simulink model "Project_template"  (R2014b)
settings: Solver=ode23tb  StartTime=0.0  StopTime=600  RelTol=1e-6  AbsTol=1e-6
values from neighbouring files (symbols this model uses):
  k = 1    [testfile.m]
  K_I = 0.03    [engine_sim.m]
  K_p = 0.002    [engine_sim.m]
undefined symbols (not defined in the file or in its folder): a_0, a_1, a_2, AFs, AirStep, alpha_REF_manual, alphaEND, alphaINI, alphaST, Boost_control, C_2, C_d, c_fi, c_fr_0, c_r1, c_r2, dp_thrREF, gamma_air, KiDriver, KpDriver, KpThr, KpWg, n_0, n_1, n_2, n_cyl, N_e_manual, N_e_step, n_ig_ch, n_r, NEND, NeST, Newton, NINI, p_amb, pedEND, pedINI, pedPos_manual, pedST, q_LHV, R_air, r_c, R_exh, Raphson, rho_air, rTurb, t_0, T_0, T_amb, T_hat_bef_thr, T_hat_im, T_ic, T_t, tau_d_bc, tau_th, TiThr, TiWg, V_d, V_D, V_em ... (+10)
libraries: simulink x1
(part 1 of 2)
settings Model: ExtModeTrigMode=oneshot  ExtModeArmWhenConnect=off  ExtModeAutoUpdateStatusClock=off  Creator=peran  LastModifiedBy=nicgr354
settings DataIOCC: LimitDataPoints=off  SignalLoggingSaveFormat=ModelDataLogs  SignalLoggingName=sigsOut
settings OptimizationCC: BlockReduction=off  BooleanDataType=off  UseDivisionForNetSlopeComputation=off  ExpressionDepthLimit=2147483647  InitFltsAndDblsToZero=on  SimCompilerOptimization=off
settings DebuggingCC: SaveWithParameterizedLinksMsg=none  UnderspecifiedInitializationDetection=Classic  MergeDetectMultiDrivingBlocksExec=none  SignalResolutionControl=TryResolveAllWithWarning  SolverPrmCheckMsg=none  MultiTaskDSMMsg=warning  MultiTaskCondExecSysMsg=none  FcnCallInpInsideContextMsg=UseLocalSettings  FrameProcessingCompatibilityMsg=error  AllowSymbolicDim=off  StateNameClashWarn=warning
settings HardwareCC: TargetUnknown=on
settings RTWCC: RTWCompilerOptimization=off
settings GRTTargetCC: TargetFcnLib=ansi_tfl_tmw.mat  ModelReferenceCompliant=off  CombineOutputUpdateFcns=off  MatFileLogging=off  GRTInterface=on
settings ConfigComp: CovMetricSettings=dw  CovHtmlReporting=on  CovSaveCumulativeToWorkspaceVar=on  CovSaveSingleToWorkspaceVar=on  CovModelRefEnable=Off  CovExternalEMLEnable=off  CovSFcnEnable=off

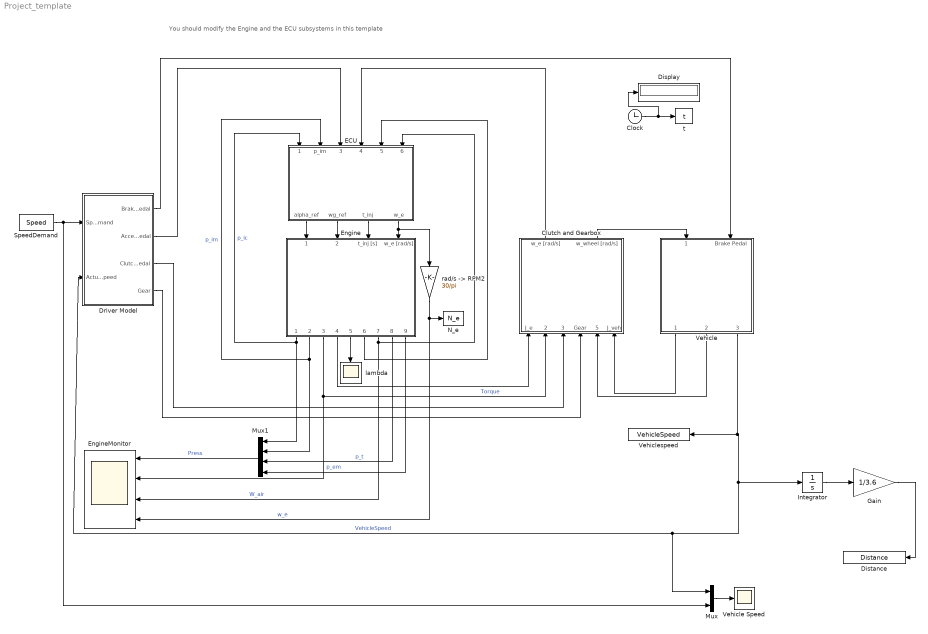
== system Project_template ==
  note: You should modify the Engine and the ECU subsystems in this template
  Clock : Clock
  Clutch and Gearbox : Subsystem
  Display : Display
  Distance : ToWorkspace  VariableName=Distance  SampleTime=-1
  Driver Model : Subsystem
  ECU : Subsystem
  Engine : Subsystem
  EngineMonitor : Scope  NumInputPorts=4
      settings: TimeRange=600  YMin=10000~-25~-8.67362e-18~900  YMax=220000~175~0.085~2900  MaxDataPoints=3000
  Gain : Gain  Gain=1/3.6
  Integrator : Integrator
  Mux : Mux  Inputs=2
  Mux1 : Mux
  N_e : ToWorkspace  VariableName=N_e  SampleTime=-1
  SpeedDemand : FromWorkspace  VariableName=Speed  SampleTime=0
  Vehicle : Subsystem
  Vehicle Speed : Scope
      settings: TimeRange=600  YMin=-20  YMax=140  MaxDataPoints=3000
  Vehiclespeed : ToWorkspace  VariableName=VehicleSpeed  SampleTime=-1
  lambda : Scope
      settings: TimeRange=100  YMin=0.996  YMax=1.005  SaveName=ScopeData2  MaxDataPoints=3000
  "rad/s -> RPM2" : Gain  Gain=30/pi  SaturateOnIntegerOverflow=on  OutDataTypeStr=Inherit: Same as input  ParamDataTypeStr=Inherit: Same as input
  t : ToWorkspace  VariableName=t  SampleTime=-1
  wires:
  Vehicle/1(Vehicle Inertia [kgm^2]) -> Clutch and Gearbox/6(J_veh)
  Vehicle/2(Vehicle Torque [Nm]) -> Clutch and Gearbox/5(Tq_veh [Nm])
  Clutch and Gearbox/2(w_wheel [rad/s]) -> Vehicle/1(Wheel Speed [rad/s])
  Vehicle/3(Vehicle Speed[km/h]) -> Integrator/1, Driver Model/2(Actual speed), Mux/1, Vehiclespeed/1  "VehicleSpeed"
  Driver Model/1(Brake Pedal) -> Vehicle/2(Brake Pedal)
  Driver Model/3(Clutch Pedal) -> Clutch and Gearbox/3(Clutch Pedal)
  Driver Model/2(Accelerator Pedal) -> ECU/3(ped_pos)
  Clutch and Gearbox/1(w_e [rad/s]) -> ECU/4(w_e [rad/s])
  SpeedDemand/1 -> Driver Model/1(Speed demand), Mux/2
  Driver Model/4(Gear) -> Clutch and Gearbox/4(Gear)
  Mux/1 -> Vehicle Speed/1
  Clock/1 -> t/1, Display/1
  Engine/7(m_dot_air [kg/s]) -> EngineMonitor/3, ECU/6(m_dot_air [kg/s])  "W_air"
  Engine/6(Lambda Disc) -> ECU/5(lambdaDisc)
  Engine/2(p_im [Pa]) -> Mux1/2, ECU/2(p_im)  "p_im"
  Engine/4(J_e [kgm^2]) -> Clutch and Gearbox/1(J_e)
  Engine/3(Tq_e [Nm]) -> EngineMonitor/2, Clutch and Gearbox/2(Tq_e [Nm])  "Torque"
  Engine/1(p_bef[Pa]) -> Mux1/1, ECU/1(p_ic [Pa])  "p_ic"
  ECU/1(alpha_ref) -> Engine/1(alpha_REF [0..1])
  ECU/2(wg_ref) -> Engine/2(wg_REF [0..1])
  Mux1/1 -> EngineMonitor/1  "Press"
  Engine/5(Lambda) -> lambda/1
  Engine/8(p_t [Pa]) -> Mux1/3  "p_t"
  Engine/9(p_em  [Pa]) -> Mux1/4  "p_em"
  ECU/4(w_e) -> Engine/4(w_e [rad/s]), "rad/s -> RPM2"/1
  "rad/s -> RPM2"/1 -> EngineMonitor/4, N_e/1  "w_e"
  ECU/3(t_inj) -> Engine/3(t_inj [s])
  Integrator/1 -> Gain/1
  Gain/1 -> Distance/1

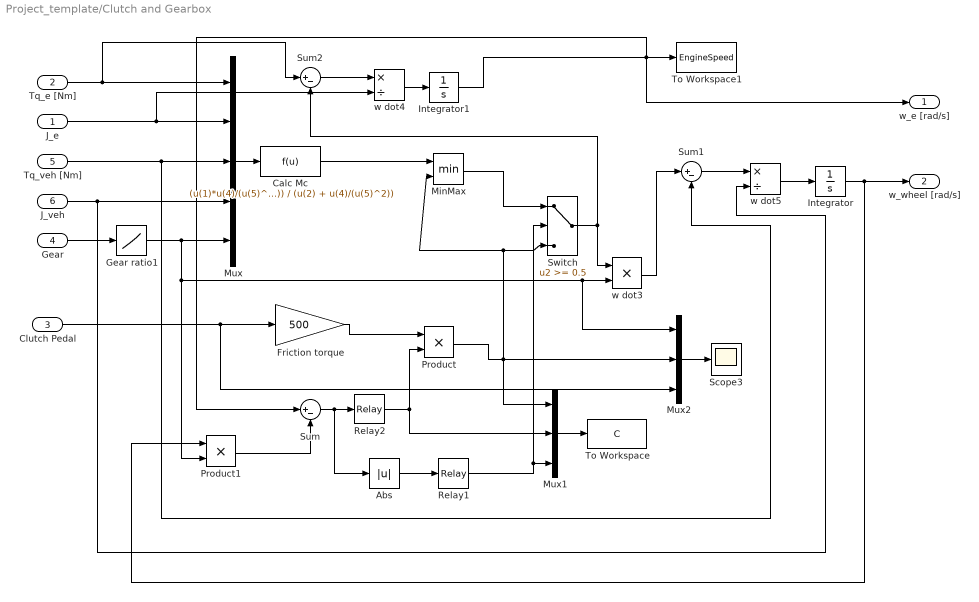
== system Project_template/Clutch and Gearbox ==
  J_e : Inport
  Tq_e [Nm] : Inport  Port=2
  Clutch Pedal : Inport  Port=3
  Gear : Inport  Port=4
  Tq_veh [Nm] : Inport  Port=5
  J_veh : Inport  Port=6
  Abs : Abs  SaturateOnIntegerOverflow=on
  Calc Mc : Fcn  Expr=(u(1)*u(4)/(u(5)^2) + u(2)*u(3)/u(5)) / (u(2) + u(4)/(u(5)^2))
  Friction torque : Gain  Gain=500  SaturateOnIntegerOverflow=on  OutDataTypeStr=Inherit: Same as input  ParamDataTypeStr=Inherit: Same as input
  Gear ratio1 : Lookup  InputValues=[0:5]  Table=[30 16 7.5 4.5 3.2 2.5]  SaturateOnIntegerOverflow=on
  Integrator : Integrator
  Integrator1 : Integrator  InitialCondition=100  LimitOutput=on  LowerSaturationLimit=100
  MinMax : MinMax  Inputs=2  SaturateOnIntegerOverflow=on  InputSameDT=on
  Mux : Mux  Inputs=5
  Mux1 : Mux  Inputs=3
  Mux2 : Mux  Inputs=3
  Product : Product  SaturateOnIntegerOverflow=on  InputSameDT=on  OutDataTypeStr=Inherit: Same as first input
  Product1 : Product  SaturateOnIntegerOverflow=on  InputSameDT=on  OutDataTypeStr=Inherit: Same as first input
  Relay1 : Relay  OnSwitchValue=10  OffSwitchValue=1e-3  OnOutputValue=0  OffOutputValue=1
  Relay2 : Relay  OnSwitchValue=1e-1  OffSwitchValue=-1e-1  OffOutputValue=-1
  Scope3 : Scope
  Sum : Sum  Inputs=|+-  SaturateOnIntegerOverflow=on  InputSameDT=on  OutDataTypeStr=Inherit: Same as first input
  Sum1 : Sum  Inputs=|+-  SaturateOnIntegerOverflow=on  InputSameDT=on  OutDataTypeStr=Inherit: Same as first input
  Sum2 : Sum  Inputs=|+-  SaturateOnIntegerOverflow=on  InputSameDT=on  OutDataTypeStr=Inherit: Same as first input
  Switch : Switch  Threshold=0.5  SaturateOnIntegerOverflow=on  InputSameDT=on
  To Workspace : ToWorkspace  VariableName=C  SaveFormat=Structure With Time  SampleTime=-1
  To Workspace1 : ToWorkspace  VariableName=EngineSpeed  SaveFormat=Structure With Time  SampleTime=-1
  w dot3 : Product  Inputs=**  SaturateOnIntegerOverflow=on  InputSameDT=on  OutDataTypeStr=Inherit: Same as first input
  w dot4 : Product  Inputs=*/  SaturateOnIntegerOverflow=on  InputSameDT=on  OutDataTypeStr=Inherit: Same as first input
  w dot5 : Product  Inputs=*/  SaturateOnIntegerOverflow=on  InputSameDT=on  OutDataTypeStr=Inherit: Same as first input
  w_e [rad/s] : Outport
  w_wheel [rad/s] : Outport  Port=2
  wires:
  Switch/1 -> w dot3/1, Sum2/2
  Relay2/1 -> Mux1/2, Product/2
  Sum/1 -> Relay2/1, Abs/1
  Abs/1 -> Relay1/1
  MinMax/1 -> Switch/1
  Calc Mc/1 -> MinMax/1
  Mux/1 -> Calc Mc/1
  Mux2/1 -> Scope3/1
  Clutch Pedal/1 -> Friction torque/1, Mux2/3
  Tq_e [Nm]/1 -> Mux/1, Sum2/1
  J_e/1 -> Mux/2, w dot4/2
  Sum2/1 -> w dot4/1
  w dot4/1 -> Integrator1/1
  Integrator1/1 -> To Workspace1/1, w_e [rad/s]/1, Sum/1
  Relay1/1 -> Mux1/3, Switch/2
  Mux1/1 -> To Workspace/1
  Product1/1 -> Sum/2
  Product/1 -> MinMax/2, Switch/3, Mux2/2, Mux1/1
  Friction torque/1 -> Product/1
  Gear/1 -> Gear ratio1/1
  Gear ratio1/1 -> Product1/2, w dot3/2, Mux2/1, Mux/5
  w dot5/1 -> Integrator/1
  Sum1/1 -> w dot5/1
  Tq_veh [Nm]/1 -> Mux/3, Sum1/2
  J_veh/1 -> Mux/4, w dot5/2
  Integrator/1 -> w_wheel [rad/s]/1, Product1/1
  w dot3/1 -> Sum1/1

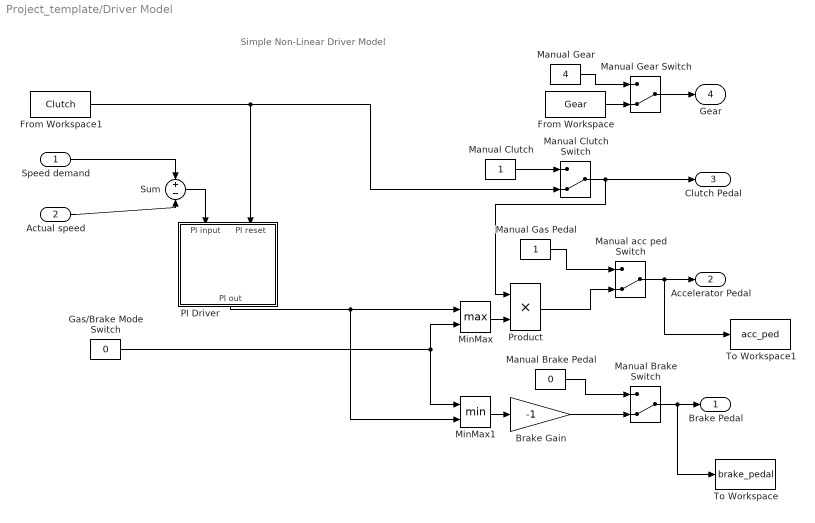
== system Project_template/Driver Model ==
  note: Simple Non-Linear Driver Model
  Speed demand : Inport
  Actual speed : Inport  Port=2
  Brake Gain : Gain  Gain=-1  SaturateOnIntegerOverflow=on  OutDataTypeStr=Inherit: Same as input  ParamDataTypeStr=Inherit: Same as input
  From Workspace : FromWorkspace  VariableName=Gear  SampleTime=0
  From Workspace1 : FromWorkspace  VariableName=Clutch  SampleTime=0  OutputAfterFinalValue=Holding final value
  Gas/Brake Mode Switch : Constant  Value=0
  Manual Clutch : Constant
  Manual Gas Pedal : Constant
  Manual Gear : Constant  Value=4
  Manual Brake Pedal : Constant  Value=0
  Manual Brake Switch : ManualSwitch  CurrentSetting=0
  Manual Clutch Switch : ManualSwitch  CurrentSetting=0
  Manual Gear Switch : ManualSwitch  CurrentSetting=0
  Manual acc ped Switch : ManualSwitch  CurrentSetting=0
  MinMax : MinMax  Function=max  Inputs=2  SaturateOnIntegerOverflow=on  InputSameDT=on
  MinMax1 : MinMax  Inputs=2  SaturateOnIntegerOverflow=on  InputSameDT=on
  PI Driver : Subsystem
  Product : Product  SaturateOnIntegerOverflow=on  InputSameDT=on  OutDataTypeStr=Inherit: Same as first input
  Sum : Sum  Inputs=+-  SaturateOnIntegerOverflow=on  InputSameDT=on  OutDataTypeStr=Inherit: Same as first input
  To Workspace : ToWorkspace  VariableName=brake_pedal  SaveFormat=Timeseries  SampleTime=-1
  To Workspace1 : ToWorkspace  VariableName=acc_ped  SaveFormat=Timeseries  SampleTime=-1
  Brake Pedal : Outport
  Accelerator Pedal : Outport  Port=2
  Clutch Pedal : Outport  Port=3
  Gear : Outport  Port=4
  wires:
  Product/1 -> Manual acc ped Switch/2
  MinMax/1 -> Product/2
  Manual acc ped Switch/1 -> To Workspace1/1, Accelerator Pedal/1
  Gas/Brake Mode Switch/1 -> MinMax1/1, MinMax/2
  MinMax1/1 -> Brake Gain/1
  PI Driver/1(PI out) -> MinMax1/2, MinMax/1
  From Workspace1/1 -> Manual Clutch Switch/2, PI Driver/2(PI reset)
  Manual Gear/1 -> Manual Gear Switch/1
  From Workspace/1 -> Manual Gear Switch/2
  Manual Gear Switch/1 -> Gear/1
  Manual Clutch/1 -> Manual Clutch Switch/1
  Brake Gain/1 -> Manual Brake Switch/2
  Manual Brake Pedal/1 -> Manual Brake Switch/1
  Manual Brake Switch/1 -> To Workspace/1, Brake Pedal/1
  Manual Clutch Switch/1 -> Clutch Pedal/1, Product/1
  Speed demand/1 -> Sum/1
  Sum/1 -> PI Driver/1(PI input)
  Actual speed/1 -> Sum/2
  Manual Gas Pedal/1 -> Manual acc ped Switch/1

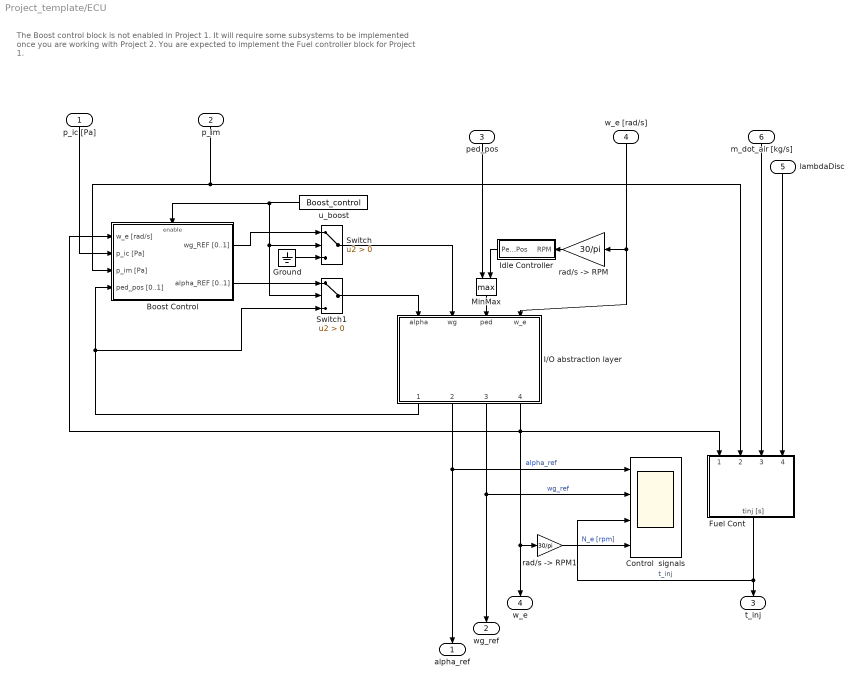
== system Project_template/ECU ==
  note: The Boost control block is not enabled in Project 1. It will require some subsystems to be
      | implemented once you are working with Project 2.
      | You are expected to implement the Fuel controller block for Project 1.
  p_ic [Pa] : Inport
  p_im : Inport  Port=2
  ped_pos : Inport  Port=3
  w_e [rad/s] : Inport  Port=4
  lambdaDisc : Inport  Port=5
  m_dot_air [kg/s] : Inport  Port=6
  Boost Control : Subsystem
  Control  signals : Scope  NumInputPorts=4
  Fuel Cont : Subsystem
  Ground : Ground
  I/O abstraction layer : Subsystem
  Idle Controller : Subsystem
  MinMax : MinMax  Function=max  Inputs=2  SaturateOnIntegerOverflow=on  InputSameDT=on
  Switch : Switch  Criteria=u2 > Threshold
  Switch1 : Switch  Criteria=u2 > Threshold
  "rad/s -> RPM" : Gain  Gain=30/pi  SaturateOnIntegerOverflow=on  OutDataTypeStr=Inherit: Same as input  ParamDataTypeStr=Inherit: Same as input
  "rad/s -> RPM1" : Gain  Gain=30/pi  SaturateOnIntegerOverflow=on  OutDataTypeStr=Inherit: Same as input  ParamDataTypeStr=Inherit: Same as input
  u_boost : Constant  Value=Boost_control
  alpha_ref : Outport
  wg_ref : Outport  Port=2
  t_inj : Outport  Port=3
  w_e : Outport  Port=4
  wires:
  Idle Controller/1(PedalPos) -> MinMax/2
  MinMax/1 -> I/O abstraction layer/3(ped)
  I/O abstraction layer/4(w_e [rad/s]) -> Fuel Cont/1(w_e [rad/s]), Boost Control/1("w_e [rad/s] "), w_e/1, "rad/s -> RPM1"/1
  w_e [rad/s]/1 -> I/O abstraction layer/4(w_e), "rad/s -> RPM"/1
  m_dot_air [kg/s]/1 -> Fuel Cont/3(m_dot_air [kg/s])
  p_ic [Pa]/1 -> Boost Control/2(p_ic [Pa])
  ped_pos/1 -> MinMax/1
  Fuel Cont/1(tinj [s]) -> Control  signals/3, t_inj/1  "t_inj"
  I/O abstraction layer/2(alpha_REF [0..1]) -> Control  signals/1, alpha_ref/1  "alpha_ref"
  I/O abstraction layer/3(wg_REF [0..100]) -> Control  signals/2, wg_ref/1  "wg_ref"
  lambdaDisc/1 -> Fuel Cont/4(lambdaDisc)
  p_im/1 -> Boost Control/3(p_im [Pa]), Fuel Cont/2(p_im [Pa])
  "rad/s -> RPM"/1 -> Idle Controller/1(RPM)
  I/O abstraction layer/1(pedPos [0..1]) -> Switch1/3, Boost Control/4(ped_pos [0..1])
  u_boost/1 -> Boost Control/Enable, Switch1/2, Switch/2
  Boost Control/2(alpha_REF [0..1]) -> Switch1/1
  Switch1/1 -> I/O abstraction layer/1(alpha)
  Switch/1 -> I/O abstraction layer/2(wg)
  Boost Control/1(wg_REF [0..1]) -> Switch/1
  Ground/1 -> Switch/3
  "rad/s -> RPM1"/1 -> Control  signals/4  "N_e [rpm]"

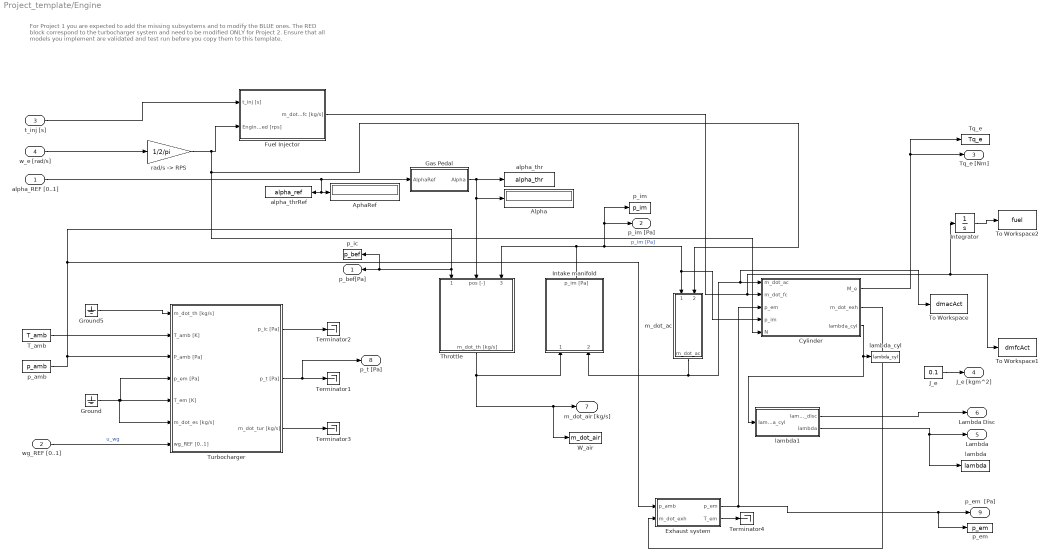
== system Project_template/Engine ==
  note: For Project 1 you are expected to add the missing subsystems and to modify the BLUE ones.
      | The RED block correspond to the turbocharger system and need to be modified ONLY for Project 2.
      | Ensure that all models you implement are validated and test run before you copy them to this template.
  alpha_REF [0..1] : Inport
  wg_REF [0..1] : Inport  Port=2
  t_inj [s] : Inport  Port=3
  w_e [rad/s] : Inport  Port=4
  Alpha : Display
  AphaRef : Display
  Cylinder : Subsystem
  Exhaust system : Subsystem
  Fuel Injector : Subsystem
  Gas Pedal : Subsystem
  Ground : Ground
  Ground5 : Ground
  Intake manifold : Subsystem
  Integrator : Integrator
  J_e : Constant  Value=0.1
  T_amb : Constant  Value=T_amb
  Terminator{1..4} (4 alike) : Terminator
  "Throttle " : Subsystem
  To Workspace : ToWorkspace  VariableName=dmacAct  SampleTime=-1
  To Workspace1 : ToWorkspace  VariableName=dmfcAct  SampleTime=-1
  To Workspace2 : ToWorkspace  VariableName=fuel  SampleTime=-1
  Tq_e : ToWorkspace  VariableName=Tq_e  SampleTime=-1
  Turbocharger : Subsystem
  W_air : ToWorkspace  VariableName=m_dot_air  SampleTime=-1
  alpha_thr : ToWorkspace  VariableName=alpha_thr  SampleTime=-1
  alpha_thrRef : ToWorkspace  VariableName=alpha_ref  SampleTime=-1
  lambda : ToWorkspace  VariableName=lambda  SampleTime=-1
  lambda1 : Subsystem
  lambda_cyl : ToWorkspace  VariableName=lambda_cyl  SampleTime=-1
  m_dot_ac : Subsystem
  p_amb : Constant  Value=p_amb
  p_em : ToWorkspace  VariableName=p_em  SampleTime=-1
  p_ic : ToWorkspace  VariableName=p_bef  SampleTime=-1
  p_im : ToWorkspace  VariableName=p_im  SampleTime=-1
  "rad/s -> RPS" : Gain  Gain=1/2/pi  SaturateOnIntegerOverflow=on  OutDataTypeStr=Inherit: Same as input  ParamDataTypeStr=Inherit: Same as input
  p_bef[Pa] : Outport
  p_im [Pa] : Outport  Port=2
  Tq_e [Nm] : Outport  Port=3
  J_e [kgm^2] : Outport  Port=4
  Lambda : Outport  Port=5
  Lambda Disc : Outport  Port=6
  m_dot_air [kg/s] : Outport  Port=7
  p_t [Pa] : Outport  Port=8
  p_em  [Pa] : Outport  Port=9
  wires:
  J_e/1 -> J_e [kgm^2]/1
  p_amb/1 -> Exhaust system/1(p_amb), "Throttle "/1(p_bef [Pa]), p_ic/1, p_bef[Pa]/1, Turbocharger/3("P_amb [Pa] ")
  Intake manifold/1(p_im [Pa]) -> p_im [Pa]/1, p_im/1, Cylinder/4(p_im), m_dot_ac/1(p_im), "Throttle "/3(p_im [Pa])  "p_im [Pa]"
  Gas Pedal/1(Alpha) -> "Throttle "/2(pos [-]), Alpha/1, alpha_thr/1
  alpha_REF [0..1]/1 -> AphaRef/1, alpha_thrRef/1, Gas Pedal/1(AlphaRef)
  w_e [rad/s]/1 -> "rad/s -> RPS"/1
  m_dot_ac/1(m_dot_ac) -> Intake manifold/2(m_dot_ac [kg/s]), To Workspace/1, Cylinder/1(m_dot_ac)
  T_amb/1 -> Turbocharger/2(T_amb [K])
  Ground/1 -> Turbocharger/6(m_dot_es [kg/s]), Turbocharger/5(T_em [K]), Turbocharger/4(p_em [Pa])
  lambda1/2(lambda) -> lambda/1, Lambda/1
  lambda1/1(lambda_bc_disc) -> Lambda Disc/1
  Exhaust system/1(p_em) -> p_em/1, p_em  [Pa]/1, Cylinder/3(p_em)
  t_inj [s]/1 -> Fuel Injector/1(t_inj [s])
  "Throttle "/1(m_dot_th [kg/s]) -> W_air/1, m_dot_air [kg/s]/1, Intake manifold/1(m_dot_th [kg/s])
  Ground5/1 -> Turbocharger/1(m_dot_th [kg/s])
  wg_REF [0..1]/1 -> Turbocharger/7(wg_REF [0..1])  "u_wg"
  Turbocharger/3(m_dot_tur [kg/s]) -> Terminator3/1
  Turbocharger/1(p_ic [Pa]) -> Terminator2/1
  Turbocharger/2(p_t [Pa]) -> p_t [Pa]/1, Terminator1/1
  "rad/s -> RPS"/1 -> Cylinder/5(N), m_dot_ac/2(Engine speed [rps]), Fuel Injector/2(Engine Speed [rps])
  Fuel Injector/1(m_dot_fc [kg/s]) -> Integrator/1, To Workspace1/1, Cylinder/2(m_dot_fc)
  Cylinder/2(m_dot_exh) -> Exhaust system/2(m_dot_exh)
  Cylinder/3(lambda_cyl) -> lambda_cyl/1, lambda1/1(lambda_cyl)
  Exhaust system/2(T_em) -> Terminator4/1
  Cylinder/1(M_e) -> Tq_e [Nm]/1, Tq_e/1
  Integrator/1 -> To Workspace2/1

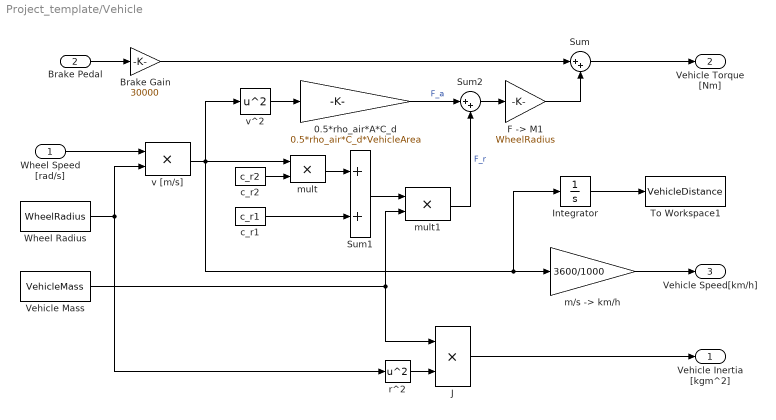
== system Project_template/Vehicle ==
  Wheel Speed [rad/s] : Inport
  Brake Pedal : Inport  Port=2
  0.5*rho_air*A*C_d : Gain  Gain=0.5*rho_air*C_d*VehicleArea  SaturateOnIntegerOverflow=on  OutDataTypeStr=Inherit: Same as input  ParamDataTypeStr=Inherit: Same as input
  Brake Gain : Gain  Gain=30000  SaturateOnIntegerOverflow=on  OutDataTypeStr=Inherit: Same as input  ParamDataTypeStr=Inherit: Same as input
  "F -> M1" : Gain  Gain=WheelRadius  SaturateOnIntegerOverflow=on  OutDataTypeStr=Inherit: Same as input  ParamDataTypeStr=Inherit: Same as input
  Integrator : Integrator
  J : Product  SaturateOnIntegerOverflow=on  OutDataTypeStr=Inherit: Same as first input
  Sum : Sum  Inputs=|++  SaturateOnIntegerOverflow=on
  Sum1 : Sum  SaturateOnIntegerOverflow=on
  Sum2 : Sum  Inputs=|++  SaturateOnIntegerOverflow=on
  To Workspace1 : ToWorkspace  VariableName=VehicleDistance  SampleTime=-1
  Vehicle Mass : Constant  Value=VehicleMass
  Wheel Radius : Constant  Value=WheelRadius
  c_r1 : Constant  Value=c_r1
  c_r2 : Constant  Value=c_r2
  "m/s -> km/h" : Gain  Gain=3600/1000  SaturateOnIntegerOverflow=on  OutDataTypeStr=Inherit: Same as input  ParamDataTypeStr=Inherit: Same as input
  mult : Product  SaturateOnIntegerOverflow=on  OutDataTypeStr=Inherit: Same as first input
  mult1 : Product  SaturateOnIntegerOverflow=on  OutDataTypeStr=Inherit: Same as first input
  r^2 : Math  Operator=square  SaturateOnIntegerOverflow=on
  v [m/s] : Product  SaturateOnIntegerOverflow=on  OutDataTypeStr=Inherit: Same as first input
  v^2 : Math  Operator=square  SaturateOnIntegerOverflow=on
  Vehicle Inertia [kgm^2] : Outport
  Vehicle Torque [Nm] : Outport  Port=2
  Vehicle Speed[km/h] : Outport  Port=3
  wires:
  Brake Pedal/1 -> Brake Gain/1
  Wheel Radius/1 -> v [m/s]/2, r^2/1
  v [m/s]/1 -> Integrator/1, "m/s -> km/h"/1, mult/1, v^2/1
  "m/s -> km/h"/1 -> Vehicle Speed[km/h]/1
  Brake Gain/1 -> Sum/1
  Sum/1 -> Vehicle Torque [Nm]/1
  r^2/1 -> J/2
  Vehicle Mass/1 -> mult1/2, J/1
  J/1 -> Vehicle Inertia [kgm^2]/1
  Integrator/1 -> To Workspace1/1
  Wheel Speed [rad/s]/1 -> v [m/s]/1
  c_r2/1 -> mult/2
  mult/1 -> Sum1/1
  c_r1/1 -> Sum1/2
  Sum1/1 -> mult1/1
  mult1/1 -> Sum2/2  "F_r"
  v^2/1 -> 0.5*rho_air*A*C_d/1
  0.5*rho_air*A*C_d/1 -> Sum2/1  "F_a"
  Sum2/1 -> "F -> M1"/1
  "F -> M1"/1 -> Sum/2

== system Project_template/Driver Model/PI Driver ==
  PI input : Inport
  PI reset : Inport  Port=2
  Integrator : Integrator  ExternalReset=either  LimitOutput=on  UpperSaturationLimit=30  LowerSaturationLimit=0
  Ki : Gain  Gain=KiDriver  SaturateOnIntegerOverflow=on  OutDataTypeStr=Inherit: Same as input  ParamDataTypeStr=Inherit: Same as input
  Kp : Gain  Gain=KpDriver  SaturateOnIntegerOverflow=on  OutDataTypeStr=Inherit: Same as input  ParamDataTypeStr=Inherit: Same as input
  Saturation : Saturate  UpperLimit=1  LowerLimit=-1
  Sum : Sum  Inputs=|++  SaturateOnIntegerOverflow=on  InputSameDT=on  OutDataTypeStr=Inherit: Same as first input
  PI out : Outport
  wires:
  PI input/1 -> Kp/1, Integrator/1
  Integrator/1 -> Ki/1
  Ki/1 -> Sum/2
  Sum/1 -> Saturation/1
  Saturation/1 -> PI out/1
  PI reset/1 -> Integrator/2
  Kp/1 -> Sum/1

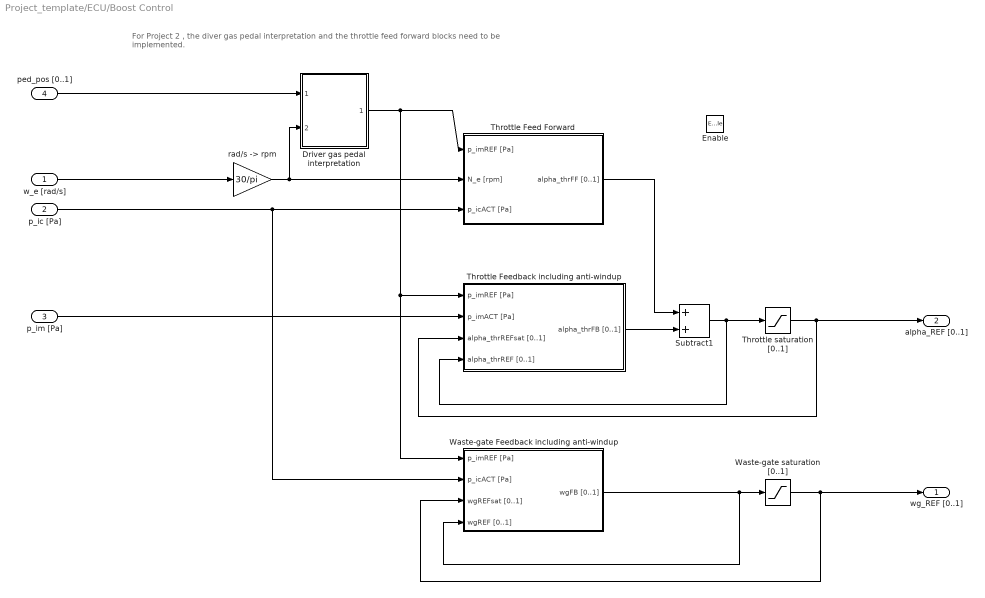
== system Project_template/ECU/Boost Control ==
  note: For Project 2 , the diver gas pedal interpretation and the throttle feed forward blocks need to be implemented.
  "w_e [rad/s] " : Inport
  p_ic [Pa] : Inport  Port=2
  p_im [Pa] : Inport  Port=3
  ped_pos [0..1] : Inport  Port=4
  Enable : EnablePort
  Driver gas pedal interpretation : Subsystem
  Subtract1 : Sum
  Throttle saturation [0..1] : Saturate  UpperLimit=1  LowerLimit=0
  Throttle Feed Forward : Subsystem
  Throttle Feedback including anti-windup : Subsystem
  Waste-gate saturation [0..1] : Saturate  UpperLimit=1  LowerLimit=0
  Waste-gate Feedback including anti-windup : Subsystem
  "rad/s -> rpm" : Gain  Gain=30/pi  SaturateOnIntegerOverflow=on  OutDataTypeStr=Inherit: Same as input  ParamDataTypeStr=Inherit: Same as input
  wg_REF [0..1] : Outport
  alpha_REF [0..1] : Outport  Port=2
  wires:
  Driver gas pedal interpretation/1(p_im_ref) -> Throttle Feed Forward/1(p_imREF [Pa]), Waste-gate Feedback including anti-windup/1(p_imREF [Pa]), Throttle Feedback including anti-windup/1(p_imREF [Pa])
  Throttle Feed Forward/1(alpha_thrFF [0..1]) -> Subtract1/1
  Throttle Feedback including anti-windup/1(alpha_thrFB [0..1]) -> Subtract1/2
  Subtract1/1 -> Throttle saturation [0..1]/1, Throttle Feedback including anti-windup/4(alpha_thrREF [0..1])
  "rad/s -> rpm"/1 -> Throttle Feed Forward/2(N_e [rpm]), Driver gas pedal interpretation/2(N_e [rpm])
  Throttle saturation [0..1]/1 -> alpha_REF [0..1]/1, Throttle Feedback including anti-windup/3(alpha_thrREFsat [0..1])
  Waste-gate saturation [0..1]/1 -> Waste-gate Feedback including anti-windup/3(wgREFsat [0..1]), wg_REF [0..1]/1
  Waste-gate Feedback including anti-windup/1(wgFB [0..1]) -> Waste-gate saturation [0..1]/1, Waste-gate Feedback including anti-windup/4(wgREF [0..1])
  ped_pos [0..1]/1 -> Driver gas pedal interpretation/1(ped_pos [0..1])
  "w_e [rad/s] "/1 -> "rad/s -> rpm"/1
  p_ic [Pa]/1 -> Waste-gate Feedback including anti-windup/2(p_icACT [Pa]), Throttle Feed Forward/3(p_icACT [Pa])
  p_im [Pa]/1 -> Throttle Feedback including anti-windup/2(p_imACT [Pa])

== system Project_template/ECU/Fuel Cont ==
  note: You have to implement here your fuel controller
  w_e [rad/s] : Inport
  p_im [Pa] : Inport  Port=2
  m_dot_air [kg/s] : Inport  Port=3
  lambdaDisc : Inport  Port=4
  Air cylinder : Subsystem
  Display : Display
  Feedback : Subsystem
  Feedforward : Subsystem
  Product : Product
  Terminator2 : Terminator
  "rad/s -> RPS" : Gain  Gain=1/2/pi  SaturateOnIntegerOverflow=on  OutDataTypeStr=Inherit: Same as input  ParamDataTypeStr=Inherit: Same as input
  tinj [s] : Outport
  wires:
  p_im [Pa]/1 -> Air cylinder/2(p_im)
  w_e [rad/s]/1 -> "rad/s -> RPS"/1
  lambdaDisc/1 -> Feedback/1(lambda_disc)
  "rad/s -> RPS"/1 -> Air cylinder/1(N), Feedforward/1(N)
  Feedforward/1(t_inj,n) -> Product/1, Display/1
  Air cylinder/1(m_dot_ac) -> Feedforward/2(m_dot_ac)
  m_dot_air [kg/s]/1 -> Terminator2/1
  Product/1 -> tinj [s]/1
  Feedback/1(F_t_inj) -> Product/2

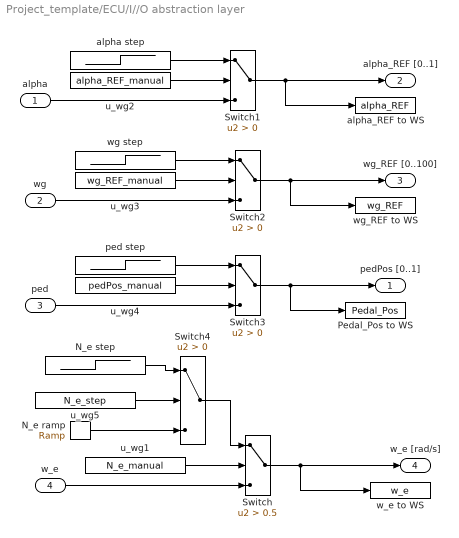
== system Project_template/ECU/I//O abstraction layer ==
  alpha : Inport
  wg : Inport  Port=2
  ped : Inport  Port=3
  w_e : Inport  Port=4
  N_e ramp : simulink/Sources/Ramp  slope=1  start=0  X0=0
  N_e step : Step  Time=NeST  Before=NINI*pi/30  After=NEND*pi/30  SampleTime=0
  Pedal_Pos to WS : ToWorkspace  VariableName=Pedal_Pos  SampleTime=-1
  Switch : Switch  Criteria=u2 > Threshold  Threshold=0.5
  Switch{1..4} (4 alike) : Switch  Criteria=u2 > Threshold
  alpha step : Step  Time=alphaST  Before=alphaINI  After=alphaEND  SampleTime=0
  alpha_REF to WS : ToWorkspace  VariableName=alpha_REF  SampleTime=-1
  ped step : Step  Time=pedST  Before=pedINI  After=pedEND  SampleTime=0
  u_wg1 : Constant  Value=N_e_manual
  u_wg2 : Constant  Value=alpha_REF_manual
  u_wg3 : Constant  Value=wg_REF_manual
  u_wg4 : Constant  Value=pedPos_manual
  u_wg5 : Constant  Value=N_e_step
  w_e to WS : ToWorkspace  VariableName=w_e  SampleTime=-1
  wg step : Step  Time=wgST  Before=wgINI  After=wgEND  SampleTime=0
  wg_REF to WS : ToWorkspace  VariableName=wg_REF  SampleTime=-1
  pedPos [0..1] : Outport
  alpha_REF [0..1] : Outport  Port=2
  wg_REF [0..100] : Outport  Port=3
  w_e [rad/s] : Outport  Port=4
  wires:
  Switch/1 -> w_e [rad/s]/1, w_e to WS/1
  u_wg1/1 -> Switch/2
  w_e/1 -> Switch/3
  Switch1/1 -> alpha_REF [0..1]/1, alpha_REF to WS/1
  alpha step/1 -> Switch1/1
  u_wg2/1 -> Switch1/2
  alpha/1 -> Switch1/3
  Switch2/1 -> wg_REF [0..100]/1, wg_REF to WS/1
  wg step/1 -> Switch2/1
  u_wg3/1 -> Switch2/2
  wg/1 -> Switch2/3
  Switch3/1 -> pedPos [0..1]/1, Pedal_Pos to WS/1
  ped step/1 -> Switch3/1
  u_wg4/1 -> Switch3/2
  ped/1 -> Switch3/3
  N_e step/1 -> Switch4/1
  Switch4/1 -> Switch/1
  N_e ramp/1 -> Switch4/3
  u_wg5/1 -> Switch4/2

== system Project_template/ECU/Idle Controller ==
  RPM : Inport
  Constant : Constant  Value=800
  Gain : Gain  Gain=1/40000  SaturateOnIntegerOverflow=on  OutDataTypeStr=Inherit: Same as input  ParamDataTypeStr=Inherit: Same as input
  Saturation : Saturate  UpperLimit=1  LowerLimit=0
  Sum : Sum  Inputs=-+  SaturateOnIntegerOverflow=on  InputSameDT=on  OutDataTypeStr=Inherit: Same as first input
  PedalPos : Outport
  wires:
  RPM/1 -> Sum/1
  Constant/1 -> Sum/2
  Saturation/1 -> PedalPos/1
  Gain/1 -> Saturation/1
  Sum/1 -> Gain/1

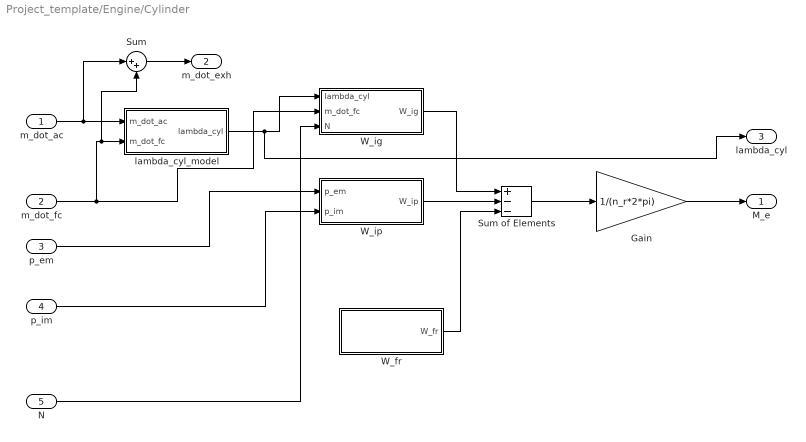
== system Project_template/Engine/Cylinder ==
  m_dot_ac : Inport
  m_dot_fc : Inport  Port=2
  p_em : Inport  Port=3
  p_im : Inport  Port=4
  N : Inport  Port=5
  Gain : Gain  Gain=1/(n_r*2*pi)
  Sum : Sum  Inputs=|++
  Sum of Elements : Sum  Inputs=+--
  W_fr : Subsystem
  W_ig : Subsystem
  W_ip : Subsystem
  lambda_cyl_model : Subsystem
  M_e : Outport
  m_dot_exh : Outport  Port=2
  lambda_cyl : Outport  Port=3
  wires:
  W_fr/1(W_fr) -> Sum of Elements/3
  W_ip/1(W_ip) -> Sum of Elements/2
  W_ig/1(W_ig) -> Sum of Elements/1
  Sum of Elements/1 -> Gain/1
  m_dot_ac/1 -> Sum/1, lambda_cyl_model/1(m_dot_ac)
  m_dot_fc/1 -> W_ig/2(m_dot_fc), Sum/2, lambda_cyl_model/2(m_dot_fc)
  lambda_cyl_model/1(lambda_cyl) -> lambda_cyl/1, W_ig/1(lambda_cyl)
  p_im/1 -> W_ip/2(p_im)
  N/1 -> W_ig/3(N)
  Gain/1 -> M_e/1
  p_em/1 -> W_ip/1(p_em)
  Sum/1 -> m_dot_exh/1

== system Project_template/Engine/Exhaust system ==
  p_amb : Inport
  m_dot_exh : Inport  Port=2
  T_em_model : Subsystem
  "m_dot_amb_model " : Subsystem
  p_em_model : Subsystem
  p_em : Outport
  T_em : Outport  Port=2
  wires:
  p_amb/1 -> "m_dot_amb_model "/3(p_amb)
  p_em_model/1(p_em) -> "m_dot_amb_model "/1(p_em), p_em/1
  T_em_model/1(T_em) -> p_em_model/3(T_em), "m_dot_amb_model "/2(T_em), T_em/1
  m_dot_exh/1 -> p_em_model/2(m_dot_exh), T_em_model/1(m_dot_exh)
  "m_dot_amb_model "/1(m_dot_amb) -> p_em_model/1(m_dot_amb)

== system Project_template/Engine/Fuel Injector ==
  t_inj [s] : Inport
  Engine Speed [rps] : Inport  Port=2
  Gain : Gain  Gain=n_cyl/n_r
  Product : Product
  m_fi : Subsystem
  m_dot_fc [kg/s] : Outport
  wires:
  t_inj [s]/1 -> m_fi/1(t_inj [s])
  m_fi/1(m_fi [kg]) -> Product/2
  Engine Speed [rps]/1 -> Gain/1
  Gain/1 -> Product/1
  Product/1 -> m_dot_fc [kg/s]/1

== system Project_template/Engine/Gas Pedal ==
  note: You are expected to implement your model here!
  AlphaRef : Inport
  1/tau_th : Gain  Gain=1/tau_th  SaturateOnIntegerOverflow=on  OutDataTypeStr=Inherit: Same as input  ParamDataTypeStr=Inherit: Same as input
  Integrator : Integrator  InitialCondition=AirStep.alpha_ref(1)
  Sum : Sum  Inputs=|+-  SaturateOnIntegerOverflow=on
  Alpha : Outport
  wires:
  AlphaRef/1 -> Sum/1
  Sum/1 -> 1/tau_th/1
  Integrator/1 -> Alpha/1, Sum/2
  1/tau_th/1 -> Integrator/1

== system Project_template/Engine/Intake manifold ==
  note: You are expected to implement your model here!
  m_dot_th [kg/s] : Inport
  m_dot_ac [kg/s] : Inport  Port=2
  Gain : Gain  Gain=R_air*T_hat_im/V_im
  Integrator : Integrator  InitialCondition=p_amb
  Sum : Sum  Inputs=|+-  SaturateOnIntegerOverflow=on
  p_im [Pa] : Outport
  wires:
  m_dot_ac [kg/s]/1 -> Sum/2
  m_dot_th [kg/s]/1 -> Sum/1
  Integrator/1 -> p_im [Pa]/1
  Sum/1 -> Gain/1
  Gain/1 -> Integrator/1

== system Project_template/Engine/Throttle  ==
  note: You are expected to implement your model here!
  p_bef [Pa] : Inport
  pos [-] : Inport  Port=2
  p_im [Pa] : Inport  Port=3
  A_eff(alpha) : Subsystem
  Constant : Constant  Value=sqrt(R_air*T_hat_bef_thr)
  Divide : Product  Inputs=*/
  PI : Subsystem
  Product : Product  Inputs=3
  Psi(PI) : Subsystem
  m_dot_th [kg/s] : Outport
  wires:
  p_im [Pa]/1 -> PI/1(p_im)  "p_im"
  p_bef [Pa]/1 -> PI/2(p_bef), Divide/1  "p_bef_thr"
  pos [-]/1 -> A_eff(alpha)/1(alpha)  "alpha"
  Psi(PI)/1(Psi) -> Product/1  "Psi"
  Product/1 -> m_dot_th [kg/s]/1
  PI/1(PI) -> Psi(PI)/1(PI)
  Constant/1 -> Divide/2
  Divide/1 -> Product/2
  A_eff(alpha)/1(A_eff) -> Product/3

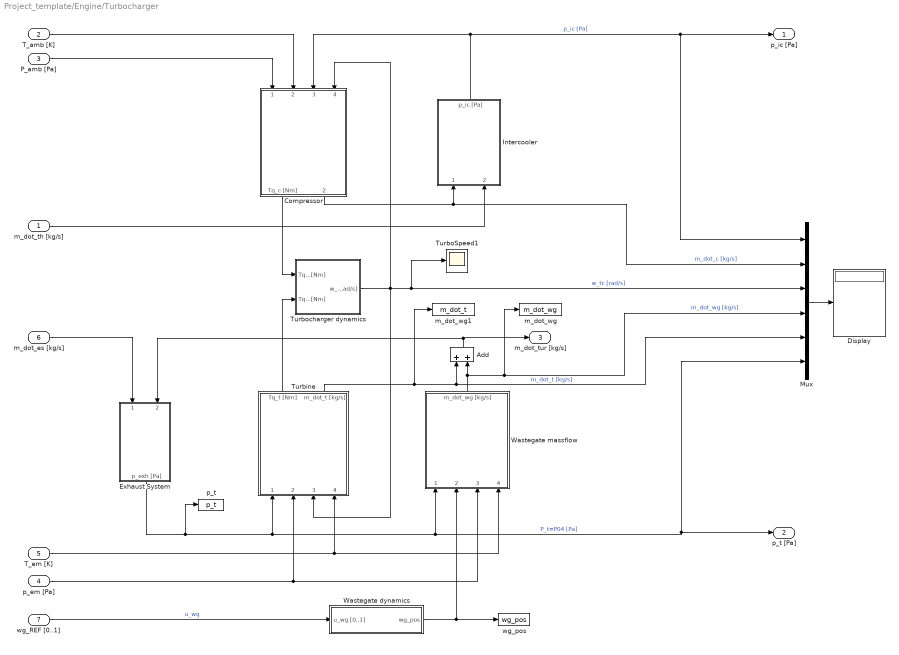
== system Project_template/Engine/Turbocharger ==
  m_dot_th [kg/s] : Inport
  T_amb [K] : Inport  Port=2
  "P_amb [Pa] " : Inport  Port=3
  p_em [Pa] : Inport  Port=4
  T_em [K] : Inport  Port=5
  m_dot_es [kg/s] : Inport  Port=6
  wg_REF [0..1] : Inport  Port=7
  Add : Sum
  Compressor : Subsystem
  Display : Display
  Exhaust System : Subsystem
  Intercooler : Subsystem
  Mux : Mux  Inputs=6
  Turbine : Subsystem
  TurboSpeed1 : Scope
  Turbocharger dynamics : Subsystem
  Wastegate dynamics : Subsystem
  Wastegate massflow : Subsystem
  m_dot_wg : ToWorkspace  VariableName=m_dot_wg  SampleTime=-1
  m_dot_wg1 : ToWorkspace  VariableName=m_dot_t  SampleTime=-1
  p_t : ToWorkspace  VariableName=p_t  SampleTime=-1
  wg_pos : ToWorkspace  VariableName=wg_pos  SampleTime=-1
  p_ic [Pa] : Outport
  p_t [Pa] : Outport  Port=2
  m_dot_tur [kg/s] : Outport  Port=3
  wires:
  Turbocharger dynamics/1(w_tc [rad/s]) -> Turbine/3(w_tc [rad/s]), Compressor/4(w_tc [rad/s]), TurboSpeed1/1, Mux/3  "w_tc [rad/s]"
  Wastegate massflow/1(m_dot_wg [kg/s]) -> m_dot_wg/1, Mux/4, Add/2  "m_dot_wg [kg/s]"
  Wastegate dynamics/1(wg_pos) -> wg_pos/1, Wastegate massflow/2(wg_pos [0..1])
  wg_REF [0..1]/1 -> Wastegate dynamics/1(u_wg [0..1])  "u_wg"
  Compressor/2(m_dot_c [kg/s]) -> Mux/2, Intercooler/1(Flow in [kg/s])  "m_dot_c [kg/s]"
  Intercooler/1(p_ic [Pa]) -> Mux/1, p_ic [Pa]/1, Compressor/3(p_c [Pa])  "p_ic [Pa]"
  Compressor/1(Tq_c [Nm]) -> Turbocharger dynamics/1(Tq_c [Nm])
  Turbine/1(Tq_t [Nm]) -> Turbocharger dynamics/2(Tq_t [Nm])
  T_amb [K]/1 -> Compressor/2(T_amb [K])
  "P_amb [Pa] "/1 -> Compressor/1(p_amb [Pa])
  m_dot_th [kg/s]/1 -> Intercooler/2(Flow  out [kg/s])
  Exhaust System/1(p_exh [Pa]) -> p_t/1, p_t [Pa]/1, Mux/6, Wastegate massflow/1(p_t [Pa]), Turbine/1("p_t [Pa] ")  "P_t=P04 [Pa]"
  p_em [Pa]/1 -> Turbine/2(p_em [Pa]), Wastegate massflow/3(p_em [Pa])
  Turbine/2(m_dot_t [kg/s]) -> m_dot_wg1/1, Mux/5, Add/1  "m_dot_t [kg/s]"
  Add/1 -> Exhaust System/2(Flow in [kg/s]), m_dot_tur [kg/s]/1
  m_dot_es [kg/s]/1 -> Exhaust System/1(Flow out [kg/s])
  Mux/1 -> Display/1
  T_em [K]/1 -> Wastegate massflow/4(T_em [K]), Turbine/4(T_em [K])

== system Project_template/Engine/lambda1 ==
  lambda_cyl : Inport
  Integrator : Integrator  InitialCondition=1
  Relay : Relay  OnSwitchValue=1  OffSwitchValue=1  OffOutputValue=-1
  Sum : Sum  Inputs=|+-
  Transport Delay : TransportDelay  DelayTime=tau_d_bc  InitialOutput=1
  lambda_bc_disc : Outport
  lambda : Outport  Port=2
  wires:
  lambda_cyl/1 -> Transport Delay/1
  Transport Delay/1 -> Sum/1
  Integrator/1 -> Sum/2, Relay/1, lambda/1
  Sum/1 -> Integrator/1
  Relay/1 -> lambda_bc_disc/1

== system Project_template/Engine/m_dot_ac ==
  p_im : Inport
  Engine speed [rps] : Inport  Port=2
  Gain : Gain  Gain=n_cyl*V_d/(n_r*R_air*T_hat_im)
  Product : Product  Inputs=3
  n_vol : Subsystem
  m_dot_ac : Outport
  wires:
  p_im/1 -> Product/1, n_vol/1(p_im)
  Engine speed [rps]/1 -> Product/3, n_vol/2(N)
  n_vol/1(n_vol) -> Product/2
  Product/1 -> Gain/1
  Gain/1 -> m_dot_ac/1

== system Project_template/ECU/Boost Control/Driver gas pedal interpretation ==
  ped_pos [0..1] : Inport
  N_e [rpm] : Inport  Port=2
  Constant : Constant
  Terminator : Terminator
  Terminator1 : Terminator
  p_im_ref : Outport
  wires:
  ped_pos [0..1]/1 -> Terminator/1
  N_e [rpm]/1 -> Terminator1/1
  Constant/1 -> p_im_ref/1

== system Project_template/ECU/Boost Control/Throttle Feed Forward ==
  p_imREF [Pa] : Inport
  N_e [rpm] : Inport  Port=2
  p_icACT [Pa] : Inport  Port=3
  Constant : Constant
  Terminator : Terminator
  Terminator1 : Terminator
  Terminator2 : Terminator
  alpha_thrFF [0..1] : Outport
  wires:
  p_imREF [Pa]/1 -> Terminator/1
  N_e [rpm]/1 -> Terminator1/1
  p_icACT [Pa]/1 -> Terminator2/1
  Constant/1 -> alpha_thrFF [0..1]/1

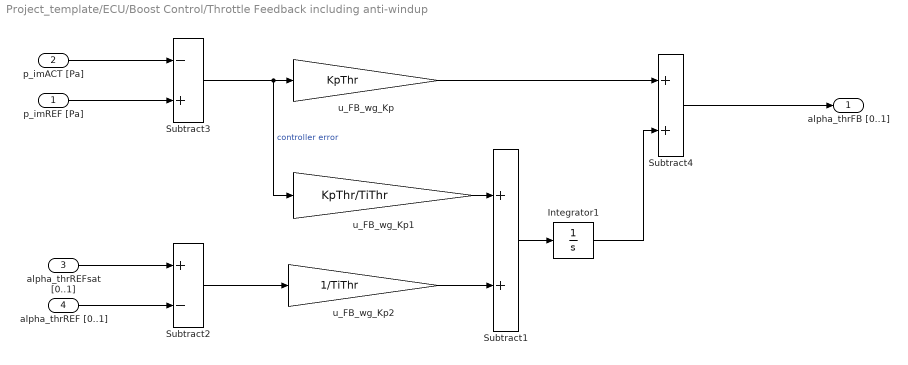
== system Project_template/ECU/Boost Control/Throttle Feedback including anti-windup ==
  p_imREF [Pa] : Inport
  p_imACT [Pa] : Inport  Port=2
  alpha_thrREFsat [0..1] : Inport  Port=3
  alpha_thrREF [0..1] : Inport  Port=4
  Integrator1 : Integrator  UpperSaturationLimit=5  LowerSaturationLimit=-5
  Subtract1 : Sum
  Subtract2 : Sum  Inputs=+-
  Subtract3 : Sum  Inputs=-+
  Subtract4 : Sum
  u_FB_wg_Kp : Gain  Gain=KpThr
  u_FB_wg_Kp1 : Gain  Gain=KpThr/TiThr
  u_FB_wg_Kp2 : Gain  Gain=1/TiThr
  alpha_thrFB [0..1] : Outport
  wires:
  p_imACT [Pa]/1 -> Subtract3/1
  p_imREF [Pa]/1 -> Subtract3/2
  Subtract3/1 -> u_FB_wg_Kp/1, u_FB_wg_Kp1/1  "controller error"
  u_FB_wg_Kp/1 -> Subtract4/1
  Subtract4/1 -> alpha_thrFB [0..1]/1
  u_FB_wg_Kp1/1 -> Subtract1/1
  alpha_thrREFsat [0..1]/1 -> Subtract2/1
  alpha_thrREF [0..1]/1 -> Subtract2/2
  Subtract2/1 -> u_FB_wg_Kp2/1
  u_FB_wg_Kp2/1 -> Subtract1/2
  Subtract1/1 -> Integrator1/1
  Integrator1/1 -> Subtract4/2

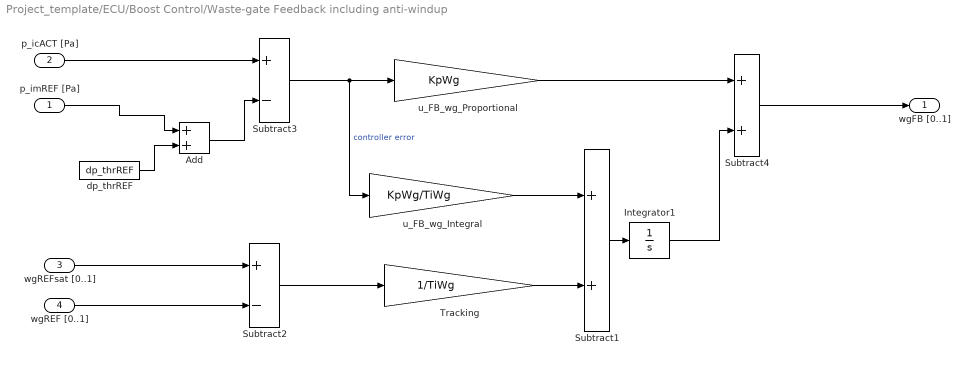
== system Project_template/ECU/Boost Control/Waste-gate Feedback including anti-windup ==
  p_imREF [Pa] : Inport
  p_icACT [Pa] : Inport  Port=2
  wgREFsat [0..1] : Inport  Port=3
  wgREF [0..1] : Inport  Port=4
  Add : Sum
  Integrator1 : Integrator
  Subtract1 : Sum
  Subtract2 : Sum  Inputs=+-
  Subtract3 : Sum  Inputs=+-
  Subtract4 : Sum
  Tracking : Gain  Gain=1/TiWg
  dp_thrREF : Constant  Value=dp_thrREF
  u_FB_wg_Integral : Gain  Gain=KpWg/TiWg
  u_FB_wg_Proportional : Gain  Gain=KpWg
  wgFB [0..1] : Outport
  wires:
  Integrator1/1 -> Subtract4/2
  Subtract1/1 -> Integrator1/1
  Tracking/1 -> Subtract1/2
  Subtract2/1 -> Tracking/1
  wgREF [0..1]/1 -> Subtract2/2
  wgREFsat [0..1]/1 -> Subtract2/1
  u_FB_wg_Integral/1 -> Subtract1/1
  Subtract4/1 -> wgFB [0..1]/1
  u_FB_wg_Proportional/1 -> Subtract4/1
  Subtract3/1 -> u_FB_wg_Proportional/1, u_FB_wg_Integral/1  "controller error"
  p_icACT [Pa]/1 -> Subtract3/1
  Add/1 -> Subtract3/2
  dp_thrREF/1 -> Add/2
  p_imREF [Pa]/1 -> Add/1

== system Project_template/ECU/Fuel Cont/Air cylinder ==
  N : Inport
  p_im : Inport  Port=2
  Gain : Gain  Gain=n_cyl*V_d/(n_r*R_air*T_hat_im)
  Product : Product  Inputs=3
  n_vol : Subsystem
  m_dot_ac : Outport
  wires:
  p_im/1 -> Product/1, n_vol/1(p_im)
  N/1 -> Product/3, n_vol/2(N)
  n_vol/1(n_vol) -> Product/2
  Product/1 -> Gain/1
  Gain/1 -> m_dot_ac/1

== system Project_template/ECU/Fuel Cont/Feedback ==
  lambda_disc : Inport
  Constant : Constant
  Gain1 : Gain  Gain=K_I
  Gain2 : Gain  Gain=K_p
  Integrator : Integrator
  Sum : Sum  Inputs=|++
  Sum1 : Sum  Inputs=|++
  F_t_inj : Outport
  wires:
  lambda_disc/1 -> Integrator/1, Gain2/1
  Integrator/1 -> Gain1/1
  Gain1/1 -> Sum/2
  Gain2/1 -> Sum/1
  Sum1/1 -> F_t_inj/1
  Sum/1 -> Sum1/1
  Constant/1 -> Sum1/2

== system Project_template/ECU/Fuel Cont/Feedforward ==
  note: m_dot_fc,n
  N : Inport
  m_dot_ac : Inport  Port=2
  Constant : Constant  Value=t_0
  Divide : Product  Inputs=*/
  Gain : Gain  Gain=1/AFs
  Gain1 : Gain  Gain=n_r/(n_cyl*c_fi)
  Sum : Sum  Inputs=|++
  t_inj,n : Outport
  wires:
  m_dot_ac/1 -> Gain/1
  Gain/1 -> Divide/1
  N/1 -> Divide/2
  Divide/1 -> Gain1/1
  Gain1/1 -> Sum/1
  Sum/1 -> t_inj,n/1
  Constant/1 -> Sum/2

== system Project_template/Engine/Cylinder/W_fr ==
  Constant : Constant  Value=c_fr_0*V_D
  W_fr : Outport
  wires:
  Constant/1 -> W_fr/1

== system Project_template/Engine/Cylinder/W_ig ==
  lambda_cyl : Inport
  m_dot_fc : Inport  Port=2
  N : Inport  Port=3
  Divide : Product  Inputs=**/
  Gain : Gain  Gain=n_r*q_LHV
  eta_tilde_ig : Subsystem
  W_ig : Outport
  wires:
  lambda_cyl/1 -> eta_tilde_ig/1(lambda_cyl)
  eta_tilde_ig/1(eta_tilde_ig) -> Divide/1
  m_dot_fc/1 -> Divide/2
  N/1 -> Divide/3
  Divide/1 -> Gain/1
  Gain/1 -> W_ig/1

== system Project_template/Engine/Cylinder/W_ip ==
  p_em : Inport
  p_im : Inport  Port=2
  Gain : Gain  Gain=V_D
  Sum : Sum  Inputs=|+-
  W_ip : Outport
  wires:
  p_im/1 -> Sum/2
  p_em/1 -> Sum/1
  Gain/1 -> W_ip/1
  Sum/1 -> Gain/1

== system Project_template/Engine/Cylinder/lambda_cyl_model ==
  m_dot_ac : Inport
  m_dot_fc : Inport  Port=2
  Divide : Product  Inputs=*/
  Gain : Gain  Gain=1/AFs
  lambda_cyl : Outport
  wires:
  Divide/1 -> Gain/1
  m_dot_ac/1 -> Divide/1
  m_dot_fc/1 -> Divide/2
  Gain/1 -> lambda_cyl/1

== system Project_template/Engine/Exhaust system/T_em_model ==
  m_dot_exh : Inport
  Constant : Constant  Value=T_0
  Gain : Gain  Gain=k
  Sqrt : Sqrt  SaturateOnIntegerOverflow=on
  Sum : Sum  Inputs=|++
  T_em : Outport
  wires:
  Sqrt/1 -> Sum/1
  m_dot_exh/1 -> Gain/1
  Gain/1 -> Sqrt/1
  Constant/1 -> Sum/2
  Sum/1 -> T_em/1

== system Project_template/Engine/Exhaust system/m_dot_amb_model  ==
  p_em : Inport
  T_em : Inport  Port=2
  p_amb : Inport  Port=3
  Divide : Product  Inputs=**/
  Gain : Gain  Gain=1/(C_2*R_exh)
  Saturation : Saturate  UpperLimit=inf  LowerLimit=0
  Sqrt : Sqrt  SaturateOnIntegerOverflow=on
  Sum : Sum  Inputs=|+-
  m_dot_amb : Outport
  wires:
  p_amb/1 -> Sum/2
  Sum/1 -> Saturation/1
  T_em/1 -> Divide/3
  p_em/1 -> Divide/1, Sum/1
  Gain/1 -> Divide/2
  Divide/1 -> Sqrt/1
  Sqrt/1 -> m_dot_amb/1
  Saturation/1 -> Gain/1

== system Project_template/Engine/Exhaust system/p_em_model ==
  m_dot_amb : Inport
  m_dot_exh : Inport  Port=2
  T_em : Inport  Port=3
  Gain : Gain  Gain=R_exh/V_em
  Integrator : Integrator  InitialCondition=p_amb
  Product : Product
  Sum : Sum  Inputs=|+-
  p_em : Outport
  wires:
  m_dot_exh/1 -> Sum/1
  m_dot_amb/1 -> Sum/2
  Sum/1 -> Product/1
  T_em/1 -> Product/2
  Product/1 -> Gain/1
  Gain/1 -> Integrator/1
  Integrator/1 -> p_em/1

== system Project_template/Engine/Fuel Injector/m_fi ==
  t_inj [s] : Inport
  Sum : Sum  Inputs=|+-
  c_fi : Gain  Gain=c_fi
  t_0 [s] : Constant  Value=t_0
  m_fi [kg] : Outport
  wires:
  t_0 [s]/1 -> Sum/2
  t_inj [s]/1 -> Sum/1
  c_fi/1 -> m_fi [kg]/1
  Sum/1 -> c_fi/1

== system Project_template/Engine/Throttle /A_eff(alpha) ==
  alpha : Inport
  Product : Product
  Sum of Elements : Sum  Inputs=+++
  a_0 : Constant  Value=a_0
  a_1 : Gain  Gain=a_1
  a_2 : Gain  Gain=a_2
  A_eff : Outport
  wires:
  alpha/1 -> a_1/1, Product/2, Product/1
  Sum of Elements/1 -> A_eff/1
  Product/1 -> a_2/1
  a_1/1 -> Sum of Elements/2
  a_2/1 -> Sum of Elements/1
  a_0/1 -> Sum of Elements/3

== system Project_template/Engine/Throttle /PI ==
  p_im : Inport
  p_bef : Inport  Port=2
  Divide : Product  Inputs=*/
  PI : Outport
  wires:
  p_im/1 -> Divide/1
  p_bef/1 -> Divide/2
  Divide/1 -> PI/1

== system Project_template/Engine/Throttle /Psi(PI) ==
  PI : Inport
  (g+1)/g : Constant  Value=(gamma_air+1)/gamma_air
  2/g : Constant  Value=2/gamma_air
  2g/(g-1) : Constant  Value=(2*gamma_air)/(gamma_air-1)
  Math Function : Math  Operator=pow  SaturateOnIntegerOverflow=on
  Math Function1 : Math  Operator=pow  SaturateOnIntegerOverflow=on
  MinMax : MinMax  Function=max  Inputs=2
  PI critical (2/(g+1))^(g/(g-1)) : Constant  Value=(2/(gamma_air+1))^(gamma_air/(gamma_air-1))
  Product : Product  RndMeth=Zero
  Sqrt : Sqrt  AlgorithmType=Newton-Raphson  SaturateOnIntegerOverflow=on
  Subtract : Sum  Inputs=+-
  "[0,1]" : Saturate  UpperLimit=1  LowerLimit=0
  Psi : Outport
  wires:
  PI/1 -> "[0,1]"/1  "PI"
  PI critical (2/(g+1))^(g/(g-1))/1 -> MinMax/2
  MinMax/1 -> Math Function/1, Math Function1/1  "PIlim"
  2/g/1 -> Math Function/2
  (g+1)/g/1 -> Math Function1/2
  "[0,1]"/1 -> MinMax/1
  Math Function/1 -> Subtract/1
  Math Function1/1 -> Subtract/2
  Subtract/1 -> Product/1
  2g/(g-1)/1 -> Product/2
  Product/1 -> Sqrt/1
  Sqrt/1 -> Psi/1  "Psi"

== system Project_template/Engine/Turbocharger/Compressor ==
  note: You are expected to fill in these blocks, only for Project 2!
  p_amb [Pa] : Inport
  T_amb [K] : Inport  Port=2
  p_c [Pa] : Inport  Port=3
  w_tc [rad/s] : Inport  Port=4
  PiCmax : Subsystem
  Product4 : Product  Inputs=*/  RndMeth=Zero
  Tc : Subsystem
  Tq_c : Subsystem
  WcCorr : Subsystem
  WcCorr2Wc : Subsystem
  etaC : Subsystem
  Tq_c [Nm] : Outport
  m_dot_c [kg/s] : Outport  Port=2
  wires:
  w_tc [rad/s]/1 -> PiCmax/2(w_tc [rad/s]), Tq_c/4(w_tc)
  p_c [Pa]/1 -> Product4/1
  p_amb [Pa]/1 -> WcCorr2Wc/1(p_amb [Pa]), Product4/2
  T_amb [K]/1 -> PiCmax/1(Tamb [K]), WcCorr2Wc/2(T_amb [K]), Tc/3(Tamb [K]), Tq_c/3(Tamb)
  WcCorr2Wc/1(m_dot_c  [Kg/s]) -> m_dot_c [kg/s]/1, Tq_c/1(m_dot_c)
  Product4/1 -> WcCorr/2(PiC), etaC/2(PiC), Tc/2(PiC)  "PiC"
  PiCmax/1(PiCmax) -> WcCorr/1(PiCmax)
  WcCorr/1(m_dot_cCorr) -> WcCorr2Wc/3(m_dot_cCorr), etaC/1(m_dot_cCorr)
  etaC/1(etaC) -> Tc/1(etaC)
  Tc/1(Tc [Nm]) -> Tq_c/2(Tc)
  Tq_c/1(Tq_c) -> Tq_c [Nm]/1

== system Project_template/Engine/Turbocharger/Exhaust System ==
  Flow out [kg/s] : Inport
  Flow in [kg/s] : Inport  Port=2
  Integrator : Integrator  InitialCondition=103e3
  Product : Product  Inputs=***/  SaturateOnIntegerOverflow=on  OutDataTypeStr=Inherit: Same as first input
  R : Constant  Value=R_exh
  Sum : Sum  Inputs=|+-  SaturateOnIntegerOverflow=on
  T_t : Constant  Value=T_t
  V_es : Constant  Value=V_es
  p_exh [Pa] : Outport
  wires:
  V_es/1 -> Product/4
  Sum/1 -> Product/1
  T_t/1 -> Product/3
  R/1 -> Product/2
  Flow out [kg/s]/1 -> Sum/2
  Flow in [kg/s]/1 -> Sum/1
  Product/1 -> Integrator/1
  Integrator/1 -> p_exh [Pa]/1

== system Project_template/Engine/Turbocharger/Intercooler ==
  Flow in [kg/s] : Inport
  Flow  out [kg/s] : Inport  Port=2
  Integrator : Integrator  InitialCondition=p_amb  LowerSaturationLimit=0
  Product : Product  Inputs=***/  SaturateOnIntegerOverflow=on  OutDataTypeStr=Inherit: Same as first input
  R : Constant  Value=R_air
  Sum : Sum  Inputs=|+-  SaturateOnIntegerOverflow=on
  T_ic : Constant  Value=T_ic
  V_ic : Constant  Value=V_ic
  p_ic [Pa] : Outport
  wires:
  Integrator/1 -> p_ic [Pa]/1
  Flow in [kg/s]/1 -> Sum/1
  Flow  out [kg/s]/1 -> Sum/2
  R/1 -> Product/2
  T_ic/1 -> Product/3
  Sum/1 -> Product/1
  V_ic/1 -> Product/4
  Product/1 -> Integrator/1

== system Project_template/Engine/Turbocharger/Turbine ==
  note: You are expected to implement your model here, only for Project 2!
  "p_t [Pa] " : Inport
  p_em [Pa] : Inport  Port=2
  w_tc [rad/s] : Inport  Port=3
  T_em [K] : Inport  Port=4
  BSR : Subsystem
  PiT : Subsystem
  TFP2Wt : Subsystem
  TFPmod : Subsystem
  Tq_t : Subsystem
  Tt : Subsystem
  etaT : Subsystem
  Tq_t [Nm] : Outport
  m_dot_t [kg/s] : Outport  Port=2
  wires:
  w_tc [rad/s]/1 -> BSR/3(w_tc [rad/s]), Tq_t/4(w_tc [rad/s])
  "p_t [Pa] "/1 -> PiT/2(p_t)
  p_em [Pa]/1 -> PiT/1(p_em), TFP2Wt/1(p_em [Pa])
  PiT/1(PiT) -> TFPmod/1(PiT), BSR/2(PiT), Tt/3(PiT)
  TFPmod/1(TFPmod) -> TFP2Wt/2(TFP)
  TFP2Wt/1(m_dot_t [kg/s]) -> m_dot_t [kg/s]/1, Tq_t/1(m_dot_t [kg/s])
  BSR/1(BSR) -> etaT/1(BSR)
  T_em [K]/1 -> TFP2Wt/3(T_em [k]), BSR/1(T_em [K]), Tq_t/2(Tem [K]), Tt/1(Tem [K])
  etaT/1(etaT) -> Tt/2(etaT)
  Tt/1(Tt [K]) -> Tq_t/3(Tt [K])
  Tq_t/1(Tq_t [Nm]) -> Tq_t [Nm]/1

== system Project_template/Engine/Turbocharger/Turbocharger dynamics ==
  Tq_c [Nm] : Inport
  Tq_t [Nm] : Inport  Port=2
  Ground : Ground
  Terminator : Terminator
  Terminator1 : Terminator
  w_tc [rad/s] : Outport
  wires:
  Tq_t [Nm]/1 -> Terminator/1
  Tq_c [Nm]/1 -> Terminator1/1
  Ground/1 -> w_tc [rad/s]/1

== system Project_template/Engine/Turbocharger/Wastegate dynamics ==
  note: You are expected to implement your model here, only for Project 2!
  u_wg [0..1] : Inport
  Ground1 : Ground
  Terminator1 : Terminator
  wg_pos : Outport
  wires:
  u_wg [0..1]/1 -> Terminator1/1
  Ground1/1 -> wg_pos/1

== system Project_template/Engine/Turbocharger/Wastegate massflow ==
  note: You are expected to implement your model here, only for Project 2!
  p_t [Pa] : Inport
  wg_pos [0..1] : Inport  Port=2
  p_em [Pa] : Inport  Port=3
  T_em [K] : Inport  Port=4
  Divide : Product  Inputs=*/
  Ground1 : Ground
  R : Constant  Value=R_exh
  Terminator{1..4} (4 alike) : Terminator
  m_dot_wg [kg/s] : Outport
  wires:
  p_em [Pa]/1 -> Divide/2
  Divide/1 -> Terminator1/1  "PI"
  p_t [Pa]/1 -> Divide/1
  Ground1/1 -> m_dot_wg [kg/s]/1
  wg_pos [0..1]/1 -> Terminator2/1
  T_em [K]/1 -> Terminator3/1
  R/1 -> Terminator4/1  "R"

== system Project_template/Engine/m_dot_ac/n_vol ==
  p_im : Inport
  N : Inport  Port=2
  Constant : Constant  Value=n_0
  Gain : Gain  Gain=n_1
  Gain1 : Gain  Gain=n_2
  Sqrt : Sqrt  SaturateOnIntegerOverflow=on
  Sum of Elements : Sum  Inputs=+++
  n_vol : Outport
  wires:
  Sum of Elements/1 -> n_vol/1
  Constant/1 -> Sum of Elements/1
  p_im/1 -> Sqrt/1
  Sqrt/1 -> Gain/1
  Gain/1 -> Sum of Elements/2
  N/1 -> Gain1/1
  Gain1/1 -> Sum of Elements/3

== system Project_template/ECU/Fuel Cont/Air cylinder/n_vol ==
  p_im : Inport
  N : Inport  Port=2
  Constant : Constant  Value=n_0
  Gain : Gain  Gain=n_1
  Gain1 : Gain  Gain=n_2
  Sqrt : Sqrt  SaturateOnIntegerOverflow=on
  Sum of Elements : Sum  Inputs=+++
  n_vol : Outport
  wires:
  Sum of Elements/1 -> n_vol/1
  Constant/1 -> Sum of Elements/1
  p_im/1 -> Sqrt/1
  Sqrt/1 -> Gain/1
  Gain/1 -> Sum of Elements/2
  N/1 -> Gain1/1
  Gain1/1 -> Sum of Elements/3

== system Project_template/Engine/Cylinder/W_ig/eta_tilde_ig ==
  lambda_cyl : Inport
  Constant : Constant
  Gain : Gain  Gain=(1-1/r_c^(gamma_air-1))*n_ig_ch
  MinMax : MinMax  Inputs=2
  eta_tilde_ig : Outport
  wires:
  lambda_cyl/1 -> MinMax/1
  Constant/1 -> MinMax/2
  MinMax/1 -> Gain/1
  Gain/1 -> eta_tilde_ig/1

== system Project_template/Engine/Turbocharger/Compressor/PiCmax ==
  Tamb [K] : Inport
  w_tc [rad/s] : Inport  Port=2
  Ground1 : Ground
  Terminator1 : Terminator
  Terminator2 : Terminator
  PiCmax : Outport
  wires:
  w_tc [rad/s]/1 -> Terminator1/1
  Tamb [K]/1 -> Terminator2/1
  Ground1/1 -> PiCmax/1

== system Project_template/Engine/Turbocharger/Compressor/Tc ==
  etaC : Inport
  PiC : Inport  Port=2
  Tamb [K] : Inport  Port=3
  Ground1 : Ground
  Terminator1 : Terminator
  Terminator2 : Terminator
  Terminator3 : Terminator
  Tc [Nm] : Outport
  wires:
  PiC/1 -> Terminator1/1
  Tamb [K]/1 -> Terminator2/1
  etaC/1 -> Terminator3/1
  Ground1/1 -> Tc [Nm]/1

== system Project_template/Engine/Turbocharger/Compressor/Tq_c ==
  m_dot_c : Inport
  Tc : Inport  Port=2
  Tamb : Inport  Port=3
  w_tc : Inport  Port=4
  Ground1 : Ground
  Terminator{1..4} (4 alike) : Terminator
  Tq_c : Outport
  wires:
  Tamb/1 -> Terminator3/1
  w_tc/1 -> Terminator4/1
  m_dot_c/1 -> Terminator1/1
  Tc/1 -> Terminator2/1
  Ground1/1 -> Tq_c/1

== system Project_template/Engine/Turbocharger/Compressor/WcCorr ==
  PiCmax : Inport
  PiC : Inport  Port=2
  Ground1 : Ground
  Terminator1 : Terminator
  Terminator2 : Terminator
  m_dot_cCorr : Outport
  wires:
  PiCmax/1 -> Terminator1/1
  PiC/1 -> Terminator2/1
  Ground1/1 -> m_dot_cCorr/1

== system Project_template/Engine/Turbocharger/Compressor/WcCorr2Wc ==
  p_amb [Pa] : Inport
  T_amb [K] : Inport  Port=2
  m_dot_cCorr : Inport  Port=3
  Ground1 : Ground
  Terminator1 : Terminator
  Terminator2 : Terminator
  Terminator3 : Terminator
  m_dot_c  [Kg/s] : Outport
  wires:
  m_dot_cCorr/1 -> Terminator1/1
  p_amb [Pa]/1 -> Terminator2/1
  T_amb [K]/1 -> Terminator3/1
  Ground1/1 -> m_dot_c  [Kg/s]/1

== system Project_template/Engine/Turbocharger/Compressor/etaC ==
  m_dot_cCorr : Inport
  PiC : Inport  Port=2
  Ground1 : Ground
  Max : MinMax  Function=max  Inputs=2
  Terminator1 : Terminator
  Terminator2 : Terminator
  etaCmin : Constant  Value=0.2
  etaC : Outport
  wires:
  etaCmin/1 -> Max/2
  Max/1 -> etaC/1
  m_dot_cCorr/1 -> Terminator1/1
  PiC/1 -> Terminator2/1
  Ground1/1 -> Max/1

== system Project_template/Engine/Turbocharger/Turbine/BSR ==
  T_em [K] : Inport
  PiT : Inport  Port=2
  w_tc [rad/s] : Inport  Port=3
  Ground1 : Ground
  Product : Product  RndMeth=Zero
  Terminator1 : Terminator
  Terminator2 : Terminator
  Terminator3 : Terminator
  rTurb : Constant  Value=rTurb
  BSR : Outport
  wires:
  rTurb/1 -> Product/2
  w_tc [rad/s]/1 -> Product/1
  Product/1 -> Terminator1/1  "U2"
  T_em [K]/1 -> Terminator3/1
  PiT/1 -> Terminator2/1
  Ground1/1 -> BSR/1

== system Project_template/Engine/Turbocharger/Turbine/PiT ==
  p_em : Inport
  p_t : Inport  Port=2
  MinMax : MinMax  Function=max  Inputs=2
  Product4 : Product  Inputs=*/  RndMeth=Zero
  one1 : Constant
  PiT : Outport
  wires:
  Product4/1 -> MinMax/1
  one1/1 -> MinMax/2
  p_em/1 -> Product4/1
  MinMax/1 -> PiT/1  "PiT"
  p_t/1 -> Product4/2

== system Project_template/Engine/Turbocharger/Turbine/TFP2Wt ==
  p_em [Pa] : Inport
  TFP : Inport  Port=2
  T_em [k] : Inport  Port=3
  Ground1 : Ground
  Pa2kPa : Gain  Gain=1e-3  SaturateOnIntegerOverflow=on  OutDataTypeStr=Inherit: Same as input  ParamDataTypeStr=Inherit: Same as input
  Terminator1 : Terminator
  Terminator2 : Terminator
  Terminator3 : Terminator
  m_dot_t [kg/s] : Outport
  wires:
  p_em [Pa]/1 -> Pa2kPa/1
  TFP/1 -> Terminator1/1
  Pa2kPa/1 -> Terminator2/1
  T_em [k]/1 -> Terminator3/1
  Ground1/1 -> m_dot_t [kg/s]/1

== system Project_template/Engine/Turbocharger/Turbine/TFPmod ==
  PiT : Inport
  Ground1 : Ground
  Terminator1 : Terminator
  TFPmod : Outport
  wires:
  PiT/1 -> Terminator1/1
  Ground1/1 -> TFPmod/1

== system Project_template/Engine/Turbocharger/Turbine/Tq_t ==
  m_dot_t [kg/s] : Inport
  Tem [K] : Inport  Port=2
  Tt [K] : Inport  Port=3
  w_tc [rad/s] : Inport  Port=4
  Ground1 : Ground
  Terminator{1..4} (4 alike) : Terminator
  Tq_t [Nm] : Outport
  wires:
  m_dot_t [kg/s]/1 -> Terminator1/1
  Tem [K]/1 -> Terminator2/1
  Tt [K]/1 -> Terminator3/1
  w_tc [rad/s]/1 -> Terminator4/1
  Ground1/1 -> Tq_t [Nm]/1
